simulink model "PID_RE35"  (R2018a)
settings: Solver=VariableStepAuto  StartTime=0.0  StopTime=1.5  MaxStep=0.0001  RelTol=1e-3  EnableMultiTasking=on
values from neighbouring files (symbols this model uses):
  i_max = 25.1    [Maxon_Control_BD.m]
  K_G = 1 / w_nom    (= 0.00147593455727)    [Maxon_Control_BD.m]
  Kd = contr_param (3)    [Maxon_Control_BD.m]    (also in pole_place.m = double(sol.Kd))
  Ki = contr_param (1)    [Maxon_Control_BD.m]    (also in RE_35.m = 128.205128205; pole_place.m = double(sol.Ki))
  Kii = contr_param (4)    [Maxon_Control_BD.m]    (also in pole_place.m = double(sol.Kii))
  Kp = contr_param (2)    [Maxon_Control_BD.m]    (also in RE_35.m = 165.6; pole_place.m = double(sol.Kp))
  T_nom = 0.0972    [DC_contr_ZN.m]    (also in DC_mot_TF.m; Maxon_Control_BD.m = 0.101; RE_35.m)
  u_nom = 30    [Maxon_Control_BD.m]
libraries: cstblocks x1, simulink x1
settings Model: Creator=tom  LastModifiedBy=manfred
settings DataIOCC: SaveFormat=Array  SignalLoggingSaveFormat=ModelDataLogs  SaveOutput=off  SignalLogging=off  SaveTime=off
settings OptimizationCC: ExpressionDepthLimit=2147483647  InitFltsAndDblsToZero=on  LifeSpan=inf
settings DebuggingCC: UnderspecifiedInitializationDetection=Classic  MergeDetectMultiDrivingBlocksExec=none  SolverPrmCheckMsg=warning  FcnCallInpInsideContextMsg=warning  StateNameClashWarn=warning  SFUnexpectedBacktrackingDiag=warning  SFNoUnconditionalDefaultTransitionDiag=warning  SFExecutionAtInitializationDiag=none
settings HardwareCC: ProdBitPerPointer=32  ProdBitPerSizeT=32  ProdBitPerPtrDiffT=32  ProdLargestAtomicFloat=None  ProdIntDivRoundTo=Undefined  ProdEndianess=Unspecified  ProdWordSize=32  ProdHWDeviceType=32-bit Generic
settings ModelReferenceCC: PropagateSignalLabelsOutOfModel=off
settings CodeAppCC: StateflowObjectComments=on
settings GRTTargetCC: TargetLangStandard=C89/C90 (ANSI)  GeneratePreprocessorConditionals=Disable all  CombineOutputUpdateFcns=off  GRTInterface=on
settings ConfigComp: CovMetricSettings=dw  CovHtmlReporting=on  CovSaveCumulativeToWorkspaceVar=on  CovSaveSingleToWorkspaceVar=on  CovExternalEMLEnable=off  CovSFcnEnable=off

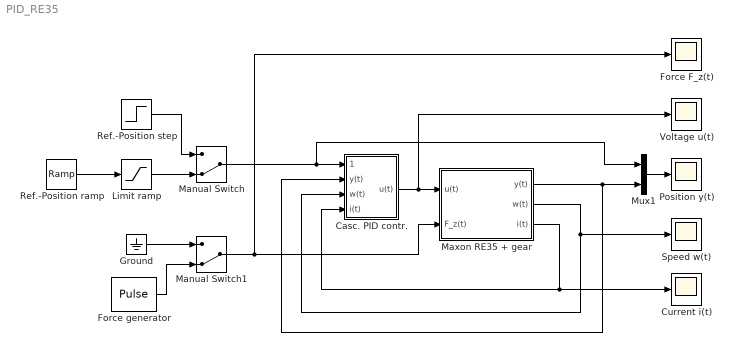
== system PID_RE35 ==
  Casc. PID contr. : Subsystem
  Current i(t) : Scope
  Force F_z(t) : Scope
  Force generator : DiscretePulseGenerator  PulseType=Time based  Amplitude=T_nom/K_G  Period=1  PulseWidth=50  PhaseDelay=1
  Ground : Ground
  Limit ramp : Saturate  LowerLimit=0
  Manual Switch : ManualSwitch  CurrentSetting=0
  Manual Switch1 : ManualSwitch  CurrentSetting=0
  Maxon RE35 + gear : Subsystem
  Mux1 : Mux  Inputs=2
  Position y(t) : Scope
  Ref.-Position ramp : simulink/Sources/Ramp  slope=1  start=0  InitialOutput=0
  Ref.-Position step : Step  Time=0  SampleTime=0
  Speed w(t) : Scope
  Voltage u(t) : Scope
  wires:
  Maxon RE35 + gear/1(y(t)) -> Mux1/2, Casc. PID contr./2(y(t))
  Maxon RE35 + gear/2(w(t)) -> Speed w(t)/1, Casc. PID contr./3(w(t))
  Maxon RE35 + gear/3(i(t)) -> Current i(t)/1, Casc. PID contr./4(i(t))
  Casc. PID contr./1(u(t)) -> Voltage u(t)/1, Maxon RE35 + gear/1(u(t))
  Ref.-Position ramp/1 -> Limit ramp/1
  Limit ramp/1 -> Manual Switch/2
  Ref.-Position step/1 -> Manual Switch/1
  Ground/1 -> Manual Switch1/1
  Force generator/1 -> Manual Switch1/2
  Mux1/1 -> Position y(t)/1
  Manual Switch/1 -> Mux1/1, Casc. PID contr./1(r_set(t))
  Manual Switch1/1 -> Maxon RE35 + gear/2(F_z(t)), Force F_z(t)/1

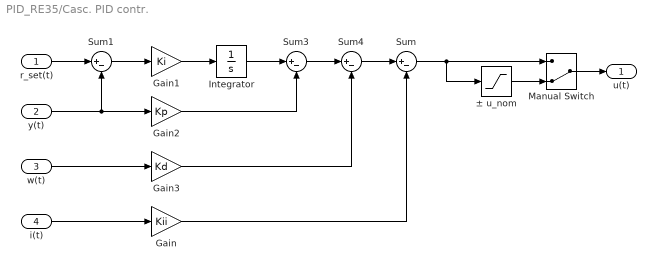
== system PID_RE35/Casc. PID contr. ==
  r_set(t) : Inport
  y(t) : Inport  Port=2
  w(t) : Inport  Port=3
  i(t) : Inport  Port=4
  Gain : Gain  Gain=Kii
  Gain1 : Gain  Gain=Ki
  Gain2 : Gain  Gain=Kp
  Gain3 : Gain  Gain=Kd
  Integrator : Integrator  LimitOutput=on  UpperSaturationLimit=60*u_nom  LowerSaturationLimit=-60*u_nom
  Manual Switch : ManualSwitch  CurrentSetting=0
  Sum{,1,3..4} (4 alike) : Sum  Inputs=|+-
  ± u_nom : Saturate  UpperLimit=u_nom  LowerLimit=-u_nom
  u(t) : Outport
  wires:
  y(t)/1 -> Gain2/1, Sum1/2
  Manual Switch/1 -> u(t)/1
  Sum/1 -> Manual Switch/1, ± u_nom/1
  Gain1/1 -> Integrator/1
  r_set(t)/1 -> Sum1/1
  Sum1/1 -> Gain1/1
  Gain/1 -> Sum/2
  w(t)/1 -> Gain3/1
  Integrator/1 -> Sum3/1
  Sum3/1 -> Sum4/1
  Gain2/1 -> Sum3/2
  Gain3/1 -> Sum4/2
  Sum4/1 -> Sum/1
  i(t)/1 -> Gain/1
  ± u_nom/1 -> Manual Switch/2

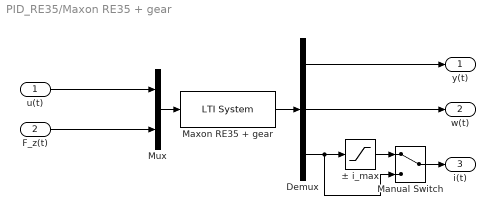
== system PID_RE35/Maxon RE35 + gear ==
  u(t) : Inport
  F_z(t) : Inport  Port=2
  Demux : Demux  Outputs=3
  Manual Switch : ManualSwitch
  Maxon RE35 + gear : cstblocks/LTI System  sys=sys  IC=[]
  Mux : Mux  Inputs=2
  ± i_max : Saturate  UpperLimit=i_max  LowerLimit=-i_max
  y(t) : Outport
  w(t) : Outport  Port=2
  i(t) : Outport  Port=3
  wires:
  Maxon RE35 + gear/1 -> Demux/1
  Demux/1 -> y(t)/1
  Demux/2 -> w(t)/1
  Demux/3 -> Manual Switch/2, ± i_max/1
  Mux/1 -> Maxon RE35 + gear/1
  u(t)/1 -> Mux/1
  F_z(t)/1 -> Mux/2
  ± i_max/1 -> Manual Switch/1
  Manual Switch/1 -> i(t)/1
